simulink model "fixed_wing_sim"  (Simulink 8.7)
settings: Solver=ode4  StartTime=0.0  StopTime=T_sim  FixedStep=ts_sim  MaxStep=10e-3  RelTol=1e-3
InitFcn:
  | % Run the initialization script
  | clear all
  | aerosonde_uav_conf_model
StopFcn:
  | %show_result
  | print_results
values from neighbouring files (symbols this model uses):
  a = param(1)    [get_field.m]    (also in print_results.m = a*scale_fac/1e3; vector_field_parameters.m = 0.85)
  AilBnd = range_ail.*degrees2rad    [aerosonde_uav_conf_model.m]
  aileron_limits = [-20*pi/180;20*pi/180]    [aerosonde_uav_conf_model.m]
  AlphaBnd = range_alpha.*degrees2rad    [aerosonde_uav_conf_model.m]
  amp_theta = amp_theta*2    [vector_field_parameters.m]
  amp_theta_c = ((1/4)*[1 1 1]/6)*U_theta*tau_theta    [vector_field_parameters.m]
  amp_v_c = [1 1 1]*(tau_v*U_v)/6    [vector_field_parameters.m]
  amp_x = [5 5 5]    [vector_field_parameters.m]
  amp_y = [5 5 5]    [vector_field_parameters.m]
  amp_z = amp_z*2    [vector_field_parameters.m]
  amp_z_c = [1 1 1]*(tau_z*U_z)/6/2    [vector_field_parameters.m]
  b = param(2)    [get_field.m]    (also in print_results.m = b*scale_fac/1e3; vector_field_parameters.m = 0.08)
  BetaBnd = range_beta.*degrees2rad    [aerosonde_uav_conf_model.m]
  Bw = 2.8956    [aerosonde_uav_conf_model.m]
  c = param(3)    [get_field.m]    (also in vector_field_parameters.m = -0.13)
  CD_0 = 0.0434    [aerosonde_uav_conf_model.m]
  CD_ail = ones(length(AlphaBnd),1)*CD_aux_ail    [aerosonde_uav_conf_model.m]
  CD_alpha_beta = zeros(length(AlphaBnd),length(BetaBnd))    [aerosonde_uav_conf_model.m]
  CD_elev = ones(length(AlphaBnd),1)*CD_aux_elev    [aerosonde_uav_conf_model.m]
  CD_mind = 0.23    [aerosonde_uav_conf_model.m]
  CD_rud = ones(length(AlphaBnd),1)*CD_aux_rud    [aerosonde_uav_conf_model.m]
  CL_0 = 0.23    [aerosonde_uav_conf_model.m]
  Cl_ail = ones(length(AlphaBnd),1)*Cl_aux_ail    [aerosonde_uav_conf_model.m]
  CL_alpha_beta = CL_alpha*ones(1,length(BetaBnd))    [aerosonde_uav_conf_model.m]
  Cl_alpha_beta = ones(length(AlphaBnd),1)*Cl_beta    [aerosonde_uav_conf_model.m]
  CL_alphadot = 1.9724    [aerosonde_uav_conf_model.m]
  CL_elev = ones(length(AlphaBnd),1)*CL_aux_elev    [aerosonde_uav_conf_model.m]
  Cl_P = ones(length(AlphaBnd),1)*Cl_aux_P    [aerosonde_uav_conf_model.m]
  CL_Q = 7.9543*QBnd    [aerosonde_uav_conf_model.m]
  Cl_R = ones(length(AlphaBnd),1)*Cl_aux_R    [aerosonde_uav_conf_model.m]
  Cl_rud = ones(length(AlphaBnd),1)*Cl_aux_rud    [aerosonde_uav_conf_model.m]
  CLE_alphat = zeros(1,length(AlphaBnd))    [aerosonde_uav_conf_model.m]
  CLE_elev = 0    [aerosonde_uav_conf_model.m]
  Cm0 = 0.135    [aerosonde_uav_conf_model.m]
  Cm_alpha_beta = Cm_alpha*ones(1,length(BetaBnd))    [aerosonde_uav_conf_model.m]
  Cm_alphadot = -10.3796    [aerosonde_uav_conf_model.m]
  Cm_elev = ones(length(AlphaBnd),1)*Cm_aux_elev    [aerosonde_uav_conf_model.m]
  Cm_Q = -38.2067*QBnd    [aerosonde_uav_conf_model.m]
  Cn_ail = ones(length(AlphaBnd),1)*Cn_aux_ail    [aerosonde_uav_conf_model.m]
  Cn_alpha_beta = ones(length(AlphaBnd),1)*Cn_beta    [aerosonde_uav_conf_model.m]
  Cn_P = ones(length(AlphaBnd),1)*Cn_aux_P    [aerosonde_uav_conf_model.m]
  Cn_R = ones(length(AlphaBnd),1)*Cn_aux_R    [aerosonde_uav_conf_model.m]
  Cn_rud = ones(length(AlphaBnd),1)*Cn_aux_rud    [aerosonde_uav_conf_model.m]
  CT_save = CT_save.*10    [aerosonde_uav_conf_model.m]    (also in helice.mat = [0.115262 0.00375054783545 -0.00666475255621 -0.006665219028)
  curve = 1    [vector_field_parameters.m]
  Cw = 0.189941    [aerosonde_uav_conf_model.m]
  CY_ail = ones(length(AlphaBnd),1)*CY_aux_ail    [aerosonde_uav_conf_model.m]
  CY_alpha_beta = ones(length(AlphaBnd),1)*CY_beta    [aerosonde_uav_conf_model.m]
  CY_P = zeros(length(AlphaBnd),length(PBnd))    [aerosonde_uav_conf_model.m]
  CY_R = zeros(length(AlphaBnd),length(RBnd))    [aerosonde_uav_conf_model.m]
  CY_rud = ones(length(AlphaBnd),1)*CY_aux_rud    [aerosonde_uav_conf_model.m]
  d = param(4)    [get_field.m]    (also in vector_field_parameters.m = -0.04)
  D_hel = 0.15    [aerosonde_uav_conf_model.m]
  d_wash = 0    [aerosonde_uav_conf_model.m]
  delta_CD = 1    [aerosonde_uav_conf_model.m]
  delta_CL = 1    [aerosonde_uav_conf_model.m]
  delta_Cl = 1    [aerosonde_uav_conf_model.m]
  delta_Cm = 1    [aerosonde_uav_conf_model.m]
  delta_Cn = 1    [aerosonde_uav_conf_model.m]
  delta_CY = 1    [aerosonde_uav_conf_model.m]
  delta_FT = 1    [aerosonde_uav_conf_model.m]
  Delta_V_EH = [ 2 1.7365 1.2985 1.0890 1.0205]    [aerosonde_uav_conf_model.m]
  Delta_V_J = [ 0 0.4 0.7 1.4 2.1]    [aerosonde_uav_conf_model.m]
  elevator_limits = [-15*pi/180;15*pi/180]    [aerosonde_uav_conf_model.m]
  ElevBnd = range_elev.*degrees2rad    [aerosonde_uav_conf_model.m]
  F_T = 19    [aerosonde_uav_conf_model.m]
  f_theta = ([5 3 1]+rand(1,3))*0.05*2*pi/freq_divisor    [vector_field_parameters.m]
  f_theta_c = ([5 3 1]+rand(1,3))*0.05*2*pi/freq_divisor    [vector_field_parameters.m]
  f_v_c = ([4 2 0.5]+rand(1,3))*0.05*2*pi/freq_divisor    [vector_field_parameters.m]
  f_x = ([6 4 2]+rand(1,3))*0.05*2*pi/freq_divisor    [vector_field_parameters.m]
  f_y = ([6 4 2]+rand(1,3))*0.05*2*pi/freq_divisor    [vector_field_parameters.m]
  f_z = ([6 4 2]+rand(1,3))*0.05*2*pi/freq_divisor    [vector_field_parameters.m]
  f_z_c = ([4 2 0.5]+rand(1,3))*0.05*2*pi/freq_divisor    [vector_field_parameters.m]
  g1 = param(5)    [get_field.m]    (also in vector_field_parameters.m = 4)
  gain_G = param(6)    [get_field.m]    (also in vector_field_parameters.m = 2.5)
  gravity = 9.807    [aerosonde_uav_conf_model.m]
  H_0 = 200    [vector_field_parameters.m]
  Heq = 200    [aerosonde_uav_conf_model.m]    (also in vector_field_parameters.m)
  induced_drag = 1/(pi*AR*osw)    (= 0.0278403324809)    [aerosonde_uav_conf_model.m]
  isTrimming = 0    [aerosonde_uav_conf_model.m]
  J_save = J_save.*1.5    [aerosonde_uav_conf_model.m]    (also in helice.mat = [0 1.22229381539 1.27367709689 1.27367940534 1.27361400442 1)
  Jx = 0.7795    [aerosonde_uav_conf_model.m]
  Jxz = 0.1211    [aerosonde_uav_conf_model.m]
  Jy = 1.122    [aerosonde_uav_conf_model.m]
  Jz = 1.752    [aerosonde_uav_conf_model.m]
  KC_h = 0.28    [aerosonde_uav_conf_model.m]
  KC_phi = -1.18    [aerosonde_uav_conf_model.m]
  KC_psi = 0.03    [aerosonde_uav_conf_model.m]
  KC_r = -0.0073    [aerosonde_uav_conf_model.m]
  KC_theta = -1.1482    [aerosonde_uav_conf_model.m]
  KC_vt = 0.9948*1    (= 0.9948)    [aerosonde_uav_conf_model.m]
  KE = -0.1562    [aerosonde_uav_conf_model.m]
  Kp = 0.18    [vector_field_parameters.m]
  KR = 0.0130    (= 0.013)    [aerosonde_uav_conf_model.m]
  Ksad = param(3)    [get_field.m]    (also in print_results.m = Ksad*scale_fac/1e3; vector_field_parameters.m = 0)
  KT = 0.0792    [aerosonde_uav_conf_model.m]
  Kv = 1    [vector_field_parameters.m]
  LIM_CENTER = LIM_CENTER*scale_fac/1e3    [print_results.m]    (also in vector_field_parameters.m = 0.2)
  M = 8.5    [aerosonde_uav_conf_model.m]    (also in print_results.m = 0)
  motor_min = 0.1    [aerosonde_uav_conf_model.m]
  motor_rate = 1    [aerosonde_uav_conf_model.m]
  p_theta = rand(1,3)*2*pi    [vector_field_parameters.m]
  p_theta_c = rand(1,3)*2*pi    [vector_field_parameters.m]
  p_v_c = rand(1,3)*2*pi    [vector_field_parameters.m]
  p_x = rand(1,3)*2*pi    [vector_field_parameters.m]
  p_y = rand(1,3)*2*pi    [vector_field_parameters.m]
  p_z = rand(1,3)*2*pi    [vector_field_parameters.m]
  p_z_c = rand(1,3)*2*pi    [vector_field_parameters.m]
  PBnd = range_P.*degrees2rad    [aerosonde_uav_conf_model.m]
  perc_int_max = 0.8    [aerosonde_uav_conf_model.m]
  phi_max = 20*pi/180    (= 0.349065850399)    [aerosonde_uav_conf_model.m]
  phi_min = -20*pi/180    (= -0.349065850399)    [aerosonde_uav_conf_model.m]
  QBnd = range_Q.*degrees2rad    [aerosonde_uav_conf_model.m]
  r = sqrt(m)    [animation.m]    (also in print_results.m)
  r_aero_abc = r_aero_struct*[-1 0 0;0 1 0;0 0 -1]    [aerosonde_uav_conf_model.m]
  r_cg_abc = r_cg_struct*[-1 0 0;0 1 0;0 0 -1]    [aerosonde_uav_conf_model.m]
  r_motor_abc = r_motor_struct*[-1 0 0;0 1 0;0 0 -1]    [aerosonde_uav_conf_model.m]
  r_tail_abc = r_aero_struct*[-1 0 0;0 1 0;0 0 -1]    [aerosonde_uav_conf_model.m]
  RBnd = range_R.*degrees2rad    [aerosonde_uav_conf_model.m]
  rho = 0.1    [aerosonde_uav_conf_model.m]
  ... (+40 more)
undefined symbols (not defined in the file or in its folder): Earth, F, Light, MIL, WGS84
libraries: aerolibwind2 x2, aerolibtransform2 x2, aerolibfltsims x1, aerolibconvert2 x1, dspsigops x1
(part 2 of 3)

== system fixed_wing_sim/A/C + Low Level Control /UAV Internal Closed Loops/UAV model/Output ==
  states : Inport
  acc : Inport  Port=2
  V_WIND : Inport  Port=3
  V_NED : Inport  Port=4
  Bus Creator : BusCreator  Inputs=11
  Bus Creator4 : BusCreator  Inputs=15
  Bus Selector : BusSelector  OutputSignals=h,theta,phi,psi,R,p_N,p_E,P,Q,R
  Bus Selector1 : BusSelector  OutputSignals=x_acc,y_acc,z_acc
  Bus Selector2 : BusSelector  OutputSignals=VT
  Bus Selector3 : BusSelector  OutputSignals=vel_N,vel_E,vel_D
  Demux : Demux  Outputs=3
  Derivative : Derivative
  Gain : Gain  Gain=180/pi
  Mux : Mux  Inputs=3
  Scope : Scope  NumInputPorts=3
  Scope1 : Scope
  Scope2 : Scope
  Terminator1 : Terminator
  Trigonometric Function : Trigonometry  Operator=atan2
  rad2deg : Gain  Gain=180/pi
  rad2deg1 : Gain  Gain=180/pi
  rad2deg2 : Gain  Gain=180/pi
  Out_model : Outport
  wires:
  states/1 -> Bus Selector/1
  acc/1 -> Bus Selector1/1
  V_WIND/1 -> Bus Selector2/1
  Bus Creator/1 -> Out_model/1
  V_NED/1 -> Bus Selector3/1
  Trigonometric Function/1 -> Bus Creator4/15, Gain/1
  Bus Selector3/1 -> Bus Creator4/7, Bus Creator/8, Mux/1, Trigonometric Function/2  "<vel_N>"
  Bus Selector3/2 -> Trigonometric Function/1, Bus Creator4/8, Bus Creator/9, Mux/2  "<vel_E>"
  Bus Selector/1 -> Bus Creator/1  "<h>"
  Bus Selector/2 -> rad2deg1/1, Bus Creator4/14, Bus Creator/2  "<theta>"
  Bus Selector/3 -> rad2deg/1, Bus Creator4/13, Bus Creator/3  "<phi>"
  Bus Selector/4 -> rad2deg2/1, Bus Creator/11, Terminator1/1  "<psi>"
  Bus Selector/5 -> Bus Creator/5  "<R>"
  Bus Selector/6 -> Scope1/1, Bus Creator/6  "<p_N>"
  Bus Selector/7 -> Bus Creator/7  "<p_E>"
  Gain/1 -> Bus Creator/4  "Psi_heading"
  Bus Selector2/1 -> Bus Creator/10  "<VT>"
  rad2deg1/1 -> Scope/1
  rad2deg/1 -> Scope/2
  rad2deg2/1 -> Scope/3
  Bus Selector1/1 -> Bus Creator4/1  "<x_acc>"
  Bus Selector1/2 -> Bus Creator4/2  "<y_acc>"
  Bus Selector1/3 -> Bus Creator4/3  "<z_acc>"
  Bus Creator4/1 -> Scope2/1
  Bus Selector/8 -> Bus Creator4/4  "<P>"
  Bus Selector/9 -> Bus Creator4/5  "<Q>"
  Bus Selector/10 -> Bus Creator4/6  "<R>"
  Bus Selector3/3 -> Mux/3, Bus Creator4/9  "<vel_D>"
  Mux/1 -> Derivative/1
  Derivative/1 -> Demux/1
  Demux/1 -> Bus Creator4/10
  Demux/2 -> Bus Creator4/11
  Demux/3 -> Bus Creator4/12

== system fixed_wing_sim/A/C + Low Level Control /UAV Internal Closed Loops/UAV model/Servos ==
  control : Inport
  Bus Creator : BusCreator  Inputs=3
  Bus Selector : BusSelector  OutputSignals=elevator,aileron,rudder,throttle
  Gain{,1..3} (4 alike) : Gain  Gain=180/pi
  Saturation : Saturate  UpperLimit=1  LowerLimit=motor_min
  Saturation1 : Saturate  UpperLimit=elevator_limits(2)  LowerLimit=elevator_limits(1)
  Saturation2 : Saturate  UpperLimit=rudder_limits(2)  LowerLimit=rudder_limits(1)
  Saturation3 : Saturate  UpperLimit=aileron_limits(2)  LowerLimit=aileron_limits(1)
  Scope : Scope  NumInputPorts=4
  angle_servos : Outport
  th_servo : Outport  Port=2
  wires:
  Saturation3/1 -> Bus Creator/2, Gain1/1  "aileron"
  Bus Creator/1 -> angle_servos/1
  Saturation1/1 -> Gain/1, Bus Creator/1  "elevator"
  Saturation2/1 -> Gain2/1, Bus Creator/3  "rudder"
  Saturation/1 -> Gain3/1, th_servo/1  "throttle"
  control/1 -> Bus Selector/1
  Bus Selector/4 -> Saturation/1  "<throttle>"
  Bus Selector/1 -> Saturation1/1  "<elevator>"
  Bus Selector/2 -> Saturation3/1  "<aileron>"
  Bus Selector/3 -> Saturation2/1  "<rudder>"
  Gain/1 -> Scope/1
  Gain3/1 -> Scope/4
  Gain2/1 -> Scope/3
  Gain1/1 -> Scope/2

== system fixed_wing_sim/A/C + Low Level Control /UAV Internal Closed Loops/UAV model/Aerodynamics Equations/F_Aero_WIND ==
  v_WIND : Inport
  servos : Inport  Port=2
  density : Inport  Port=3
  w_ABC : Inport  Port=4
  Bus Creator : BusCreator  Inputs=3
  Bus Selector : BusSelector  OutputSignals=VT,alpha,beta
  Bus Selector2 : BusSelector  OutputSignals=P,Q,R
  Drag Force : Subsystem
  Gain : Gain  Gain=-1
  Gain1 : Gain  Gain=-1
  Gain2 : Gain
  Lift Force : Subsystem
  Side Force : Subsystem
  F_WIND : Outport
  wires:
  Drag Force/1(D) -> Gain/1
  Bus Creator/1 -> F_WIND/1
  v_WIND/1 -> Bus Selector/1
  Gain/1 -> Bus Creator/1
  Bus Selector/1 -> Side Force/3(VT), Lift Force/3(VT), Drag Force/4(VT)  "<VT>"
  Bus Selector/2 -> Drag Force/1(alpha), Lift Force/1(alpha), Side Force/2(alpha)  "<alpha>"
  Side Force/1(Y) -> Gain2/1
  Gain1/1 -> Bus Creator/3
  density/1 -> Side Force/4(density), Drag Force/5(density), Lift Force/4(density)
  Bus Selector/3 -> Drag Force/2(beta), Side Force/1(beta), Lift Force/2(beta)  "<beta>"
  w_ABC/1 -> Bus Selector2/1
  Lift Force/1(L) -> Gain1/1
  Bus Selector2/1 -> Side Force/6(P)  "<P>"
  Bus Selector2/2 -> Lift Force/6(Q)  "<Q>"
  Bus Selector2/3 -> Side Force/7(R)  "<R>"
  Gain2/1 -> Bus Creator/2
  servos/1 -> Side Force/5(servos), Lift Force/5(servos), Drag Force/6(servos)
  Lift Force/2(CL) -> Drag Force/3(CL)

== system fixed_wing_sim/A/C + Low Level Control /UAV Internal Closed Loops/UAV model/Aerodynamics Equations/F_TAIL_WIND --> F_ABC ==
  note: ABC = ( R_(alpha) )^T * WIND
  v_WIND : Inport
  WIND : Inport  Port=2
  Bus Selector : BusSelector  OutputSignals=alpha_t
  Math Function : Math  Operator=transpose  SaturateOnIntegerOverflow=on
  Product1 : Product  Multiplication=Matrix(*)  RndMeth=Zero
  R_(alpha) : Subsystem
  ABC : Outport
  wires:
  v_WIND/1 -> Bus Selector/1
  WIND/1 -> Product1/2
  Product1/1 -> ABC/1
  Math Function/1 -> Product1/1
  Bus Selector/1 -> R_(alpha)/1(In1)  "<alpha_t>"
  R_(alpha)/1(Out1) -> Math Function/1

== system fixed_wing_sim/A/C + Low Level Control /UAV Internal Closed Loops/UAV model/Aerodynamics Equations/F_Tail_WIND ==
  note: Dynamic Pressure
  v_WIND : Inport
  servos : Inport  Port=2
  density : Inport  Port=3
  Delta_V_EH : Inport  Port=4
  teste_V : Inport  Port=5
  Add : Sum
  Area Empenagem : Gain  Gain=Sh
  Bus Selector : BusSelector  OutputSignals=alpha_t,VT_tail
  Bus Selector1 : BusSelector  OutputSignals=elevator
  Bus Selector2 : BusSelector  OutputSignals=VT
  CLE_alphat : Lookup  InputValues=AlphaBnd  Table=CLE_alphat
  Constant4 : Constant  Value=0
  Gain : Gain  Gain=0.5
  Gain3 : Gain  Gain=CLE_elev  SaturateOnIntegerOverflow=on  OutDataTypeStr=Inherit: Same as input  ParamDataTypeStr=Inherit: Same as input
  Math Function : Math  Operator=square  SaturateOnIntegerOverflow=on
  Mux : Mux  Inputs=3
  Product : Product  RndMeth=Zero
  Product1 : Product  RndMeth=Zero
  Product2 : Product  RndMeth=Zero
  Terminator : Terminator
  Z + down : Gain  Gain=-1
  F_Tail_WIND : Outport
  wires:
  v_WIND/1 -> Bus Selector/1
  servos/1 -> Bus Selector1/1
  Bus Selector1/1 -> Gain3/1  "<elevator>"
  Bus Selector/1 -> CLE_alphat/1  "<alpha_t>"
  Product/1 -> Gain/1
  density/1 -> Product/1
  Math Function/1 -> Product/2
  Product1/1 -> Math Function/1
  Delta_V_EH/1 -> Product1/2
  CLE_alphat/1 -> Add/1
  Gain3/1 -> Add/2
  Add/1 -> Product2/1
  Gain/1 -> Product2/2
  Product2/1 -> Area Empenagem/1
  Mux/1 -> F_Tail_WIND/1
  Area Empenagem/1 -> Z + down/1
  Z + down/1 -> Mux/3
  Constant4/1 -> Mux/1, Mux/2
  teste_V/1 -> Bus Selector2/1
  Bus Selector/2 -> Product1/1  "<VT_tail>"
  Bus Selector2/1 -> Terminator/1  "<VT>"

== system fixed_wing_sim/A/C + Low Level Control /UAV Internal Closed Loops/UAV model/Aerodynamics Equations/F_WIND --> F_ABC ==
  note: ABC = ( R_beta * R_(alpha) )^T * WIND
  v_WIND : Inport
  WIND : Inport  Port=2
  Bus Selector : BusSelector  OutputSignals=alpha,beta
  Math Function : Math  Operator=transpose  SaturateOnIntegerOverflow=on
  Product : Product  Multiplication=Matrix(*)  RndMeth=Zero
  Product1 : Product  Multiplication=Matrix(*)  RndMeth=Zero
  R_(alpha) : Subsystem
  R_beta : Subsystem
  ABC : Outport
  wires:
  R_beta/1(Out1) -> Product/1
  R_(alpha)/1(Out1) -> Product/2
  v_WIND/1 -> Bus Selector/1
  WIND/1 -> Product1/2
  Product1/1 -> ABC/1
  Product/1 -> Math Function/1
  Math Function/1 -> Product1/1
  Bus Selector/1 -> R_(alpha)/1(In1)  "<alpha>"
  Bus Selector/2 -> R_beta/1(In1)  "<beta>"

== system fixed_wing_sim/A/C + Low Level Control /UAV Internal Closed Loops/UAV model/Aerodynamics Equations/M_Aero_WIND ==
  v_WIND : Inport
  servos : Inport  Port=2
  density : Inport  Port=3
  w_ABC : Inport  Port=4
  Bus Creator : BusCreator  Inputs=3
  Bus Selector : BusSelector  OutputSignals=VT,alpha,beta
  Bus Selector2 : BusSelector  OutputSignals=P,Q,R
  Pitching Moment : Subsystem
  Rolling Moment : Subsystem
  Yawing Moment : Subsystem
  M_ABC : Outport
  wires:
  Bus Creator/1 -> M_ABC/1
  v_WIND/1 -> Bus Selector/1
  servos/1 -> Rolling Moment/7(servos), Pitching Moment/5(servo), Yawing Moment/5(servos)
  w_ABC/1 -> Bus Selector2/1
  density/1 -> Yawing Moment/4(density), Rolling Moment/4(density), Pitching Moment/4(density)
  Rolling Moment/1(Cl) -> Bus Creator/1
  Pitching Moment/1(Cm) -> Bus Creator/2
  Yawing Moment/1(Cn) -> Bus Creator/3
  Bus Selector2/1 -> Rolling Moment/5(P), Yawing Moment/6(P)  "<P>"
  Bus Selector2/2 -> Pitching Moment/6(Q)  "<Q>"
  Bus Selector2/3 -> Yawing Moment/7(R), Rolling Moment/6(R)  "<R>"
  Bus Selector/1 -> Rolling Moment/3(VT), Yawing Moment/3(VT), Pitching Moment/3(VT)  "<VT>"
  Bus Selector/3 -> Rolling Moment/1(beta), Yawing Moment/1(beta), Pitching Moment/2(beta)  "<beta>"
  Bus Selector/2 -> Rolling Moment/2(alpha), Pitching Moment/1(alpha), Yawing Moment/2(alpha)  "<alpha>"

== system fixed_wing_sim/A/C + Low Level Control /UAV Internal Closed Loops/UAV model/Aerodynamics Equations/U' V' W' --> VT,alpha,beta ==
  v_ABC : Inport
  Bus Creator : BusCreator  Inputs=3
  alpha : Fcn  Expr=atan2(u(3),u(1))
  beta : Fcn  Expr=asin(u(2)/sqrt(u(1)^2 + u(2)^2 + u(3)^2))
  vector_norm : Fcn  Expr=sqrt(u(1)^2 + u(2)^2 + u(3)^2)
  v_WIND : Outport
  wires:
  Bus Creator/1 -> v_WIND/1
  v_ABC/1 -> vector_norm/1, alpha/1, beta/1
  vector_norm/1 -> Bus Creator/1  "VT"
  alpha/1 -> Bus Creator/2  "alpha"
  beta/1 -> Bus Creator/3  "beta"

== system fixed_wing_sim/A/C + Low Level Control /UAV Internal Closed Loops/UAV model/Aerodynamics Equations/U' V' W' --> Vtail, alpha_t ==
  v_ABC : Inport
  w_ABC : Inport  Port=2
  wind : Inport  Port=3
  Add : Sum  Inputs=++-
  Bus Creator : BusCreator  Inputs=2
  Bus Selector : BusSelector  OutputSignals=U,W
  Bus Selector1 : BusSelector  OutputSignals=Q
  Bus Selector2 : BusSelector  OutputSignals=alpha,VT
  Constant1 : Constant  Value=xt
  Gain : Gain  Gain=d_wash
  Mux : Mux  Inputs=2
  Product : Product  RndMeth=Zero
  Product1 : Product  RndMeth=Zero
  VT_tail : Fcn  Expr=sqrt(u(1)^2 + u(2)^2 )
  alpha_t : Fcn  Expr=atan2(u(2),u(1))
  v_TAIL : Outport
  wires:
  Bus Creator/1 -> v_TAIL/1
  VT_tail/1 -> Bus Creator/1  "VT_tail"
  alpha_t/1 -> Bus Creator/2  "alpha_t"
  v_ABC/1 -> Bus Selector/1
  w_ABC/1 -> Bus Selector1/1
  Bus Selector1/1 -> Product/1  "<Q>"
  Constant1/1 -> Product/2
  Bus Selector/2 -> Add/1  "<W>"
  Product/1 -> Add/2
  Bus Selector/1 -> Mux/1  "<U>"
  Add/1 -> Mux/2
  Mux/1 -> VT_tail/1, alpha_t/1
  Gain/1 -> Product1/1
  wind/1 -> Bus Selector2/1
  Bus Selector2/1 -> Gain/1  "<alpha>"
  Bus Selector2/2 -> Product1/2  "<VT>"
  Product1/1 -> Add/3

== system fixed_wing_sim/A/C + Low Level Control /UAV Internal Closed Loops/UAV model/Atmosphere Model/Standard Atmosphere ==
  var_states : Inport
  g : Inport  Port=2
  Altitude Equilibrio : Constant  Value=Heq
  Bus Selector : BusSelector  OutputSignals=h
  Calc. Density : Fcn  Expr=1.225*(u(1)/288.15)^(-u(2)/(-0.0065*287.04)-1)
  Calc. Pressure : Fcn  Expr=101325*(u(1)/288.15)^(-u(2)/(-0.0065*287.04))
  Calc. Temperatura : Fcn  Expr=288.15 -0.0065*u(1)
  Function for Sound Speed : Fcn  Expr=sqrt(u*1.4*287.04)
  Mux : Mux  Inputs=2
  Mux1 : Mux  Inputs=2
  Terminator : Terminator
  rho (kg/m3) : Outport
  a (m/s) : Outport  Port=2
  T (K) : Outport  Port=3
  P (N/m2) : Outport  Port=4
  wires:
  g/1 -> Mux1/2, Mux/2
  Mux/1 -> Calc. Temperatura/1
  Mux1/1 -> Calc. Pressure/1, Calc. Density/1
  Calc. Temperatura/1 -> Mux1/1, Function for Sound Speed/1, T (K)/1  "temperature (K)"
  Calc. Pressure/1 -> P (N/m2)/1  "pressure (Pa)"
  Calc. Density/1 -> rho (kg/m3)/1  "density (Kg/m3)"
  Function for Sound Speed/1 -> a (m/s)/1  "sound speed (m/s)"
  var_states/1 -> Bus Selector/1
  Altitude Equilibrio/1 -> Terminator/1
  Bus Selector/1 -> Mux/1  "<h>"

== system fixed_wing_sim/A/C + Low Level Control /UAV Internal Closed Loops/UAV model/Body-Axes 6DOF Equations/Force Equations ==
  note: Gravity Vector in ABC
  note: Forces in ABC
  note: Term due derivative had token in NED but
      | velocity in ABC
  note: Equation: v_ABC_dot = (1/m) * F_A,T + R_ned_abc * gravity - w_ABC x v_ABC
  F_Aero_ABC : Inport
  attitude : Inport  Port=2
  F_Thrust_ABC : Inport  Port=3
  w_ABC : Inport  Port=4
  v_ABC : Inport  Port=5
  F_tail_ABC : Inport  Port=6
  Add : Sum  Inputs=+++
  Add1 : Sum  Inputs=++-
  Bus Creator : BusCreator  Inputs=3
  Demux : Demux  Outputs=3
  Mux : Mux  Inputs=3
  NED --> ABC : Subsystem
  Product : Product  RndMeth=Zero
  Vector Product : Subsystem  Description=Vector Product
  axis_X : Constant  Value=0
  axis_Y : Constant  Value=0
  axis_Z : Constant  Value=gravity
  inv_M : Constant  Value=1/M
  v_ABC_dot : Outport
  acc_x_y_z : Outport  Port=2
  wires:
  axis_X/1 -> Mux/1
  axis_Y/1 -> Mux/2
  axis_Z/1 -> Mux/3
  Mux/1 -> NED --> ABC/2(NED)
  F_Aero_ABC/1 -> Add/1
  F_Thrust_ABC/1 -> Add/2
  Add/1 -> Product/1
  inv_M/1 -> Product/2
  attitude/1 -> NED --> ABC/1(attitude)
  w_ABC/1 -> Vector Product/1(V1)
  v_ABC/1 -> Vector Product/2(V2)
  Product/1 -> Add1/1, Demux/1
  Vector Product/1(V1 x V2) -> Add1/3
  Add1/1 -> v_ABC_dot/1
  NED --> ABC/1(ABC) -> Add1/2
  Bus Creator/1 -> acc_x_y_z/1
  Demux/1 -> Bus Creator/1  "x_acc"
  Demux/2 -> Bus Creator/2  "y_acc"
  Demux/3 -> Bus Creator/3  "z_acc"
  F_tail_ABC/1 -> Add/3

== system fixed_wing_sim/A/C + Low Level Control /UAV Internal Closed Loops/UAV model/Body-Axes 6DOF Equations/Kinematic Equations ==
  note: phi_dot     = P + Q*tan(theta)*sin(phi) + R*tan(theta)*cos(phi)
      |          theta_dot =  Q*cos(phi) - R*sin(phi)
      |                           psi_dot     = (Q*sin(phi) + R*cos(phi)) / cos (theta)
  note: Relationship between angular velocity of Euler angles (phi_dot, theta_dot, psi_dot) and angular velocity of axis ABC (P,Q,R)
  attitude : Inport
  w_ABC : Inport  Port=2
  Bus Selector : BusSelector  OutputSignals=phi,theta,psi
  Bus Selector1 : BusSelector  OutputSignals=P,Q,R
  Mux : Mux  Inputs=3
  Product{,1..4,6..7} (7 alike) : Product  SaturateOnIntegerOverflow=on  OutDataTypeStr=Inherit: Same as first input
  Product5 : Product  Inputs=/*  SaturateOnIntegerOverflow=on  OutDataTypeStr=Inherit: Same as first input
  Sum1 : Sum  SaturateOnIntegerOverflow=on
  Sum2 : Sum  SaturateOnIntegerOverflow=on
  Sum3 : Sum  Inputs=+-  SaturateOnIntegerOverflow=on
  Sum4 : Sum  SaturateOnIntegerOverflow=on
  Terminator : Terminator
  cos (phi) : Trigonometry  Operator=cos
  cos (theta) : Trigonometry  Operator=cos
  sin (phi) : Trigonometry
  tan (theta) : Trigonometry  Operator=tan
  attitude_dot : Outport
  wires:
  Bus Selector/2 -> cos (theta)/1, tan (theta)/1  "<theta>"
  Bus Selector/1 -> cos (phi)/1, sin (phi)/1  "<phi>"
  sin (phi)/1 -> Product/1, Product4/1, Product6/1
  cos (phi)/1 -> Product1/1, Product3/1, Product7/1
  Product1/1 -> Sum1/1
  Product/1 -> Sum1/2
  Sum1/1 -> Product2/1
  Product2/1 -> Sum2/1
  Sum2/1 -> Mux/1
  Bus Selector/3 -> Terminator/1  "<psi>"
  Product3/1 -> Sum3/1
  w_ABC/1 -> Bus Selector1/1
  Product4/1 -> Sum3/2
  cos (theta)/1 -> Product5/1
  Product6/1 -> Sum4/1
  Product7/1 -> Sum4/2
  Sum4/1 -> Product5/2
  Sum3/1 -> Mux/2
  Product5/1 -> Mux/3
  Bus Selector1/1 -> Sum2/2  "<P>"
  Mux/1 -> attitude_dot/1
  Bus Selector1/2 -> Product/2, Product3/2, Product6/2  "<Q>"
  Bus Selector1/3 -> Product1/2, Product4/2, Product7/2  "<R>"
  tan (theta)/1 -> Product2/2
  attitude/1 -> Bus Selector/1

== system fixed_wing_sim/A/C + Low Level Control /UAV Internal Closed Loops/UAV model/Body-Axes 6DOF Equations/Moment Equations ==
  note: Term due derivative had token in NED but
      | angular velocity in ABC
  note: Equation: w_ABC_dot = J^(-1)*[ M_A,T - w_ABC x J * w_ABC ]
  note: Moments in ABC due position of motor and aerodynamics
      | forces em relação gravity center and aerodynamics moments
  M_Aero_ABC : Inport
  F_Thrust_ABC : Inport  Port=2
  w_ABC : Inport  Port=3
  F_Aero_ABC : Inport  Port=4
  F_tail_ABC : Inport  Port=5
  Add : Sum  Inputs=+-
  Add1 : Sum  Inputs=-+
  Add2 : Sum  Inputs=-+
  C.G. position : Constant  Value=r_cg_abc
  Engine position1 : Constant  Value=r_aero_abc
  Engine position2 : Constant  Value=r_tail_abc
  Inertia : Subsystem
  Inverse Inertia Matrix : Subsystem
  Motor position : Constant  Value=r_motor_abc
  Product : Product  Multiplication=Matrix(*)  SaturateOnIntegerOverflow=on  OutDataTypeStr=Inherit: Same as first input
  Product1 : Product  Multiplication=Matrix(*)  SaturateOnIntegerOverflow=on  OutDataTypeStr=Inherit: Same as first input
  Product2 : Product  Multiplication=Matrix(*)  SaturateOnIntegerOverflow=on  OutDataTypeStr=Inherit: Same as first input
  Produto Vetorial1 : Subsystem
  Produto Vetorial2 : Subsystem
  Produto Vetorial3 : Subsystem
  Produto Vetorial4 : Subsystem
  Sum2 : Sum  Inputs=++++  SaturateOnIntegerOverflow=on
  Sum3 : Sum  Inputs=|+-  SaturateOnIntegerOverflow=on
  w_ABC_dot : Outport
  wires:
  Inverse Inertia Matrix/1(inv J_b) -> Product/1, Product2/1
  Sum2/1 -> Product/2
  Product/1 -> Sum3/1
  Inertia/1(J_b) -> Product1/1
  w_ABC/1 -> Product1/2, Produto Vetorial1/1(V1)
  Product1/1 -> Produto Vetorial1/2(V2)
  Produto Vetorial1/1(V1 x V2) -> Product2/2
  Product2/1 -> Sum3/2
  Motor position/1 -> Add/1
  F_Thrust_ABC/1 -> Produto Vetorial2/2(V2)
  Sum3/1 -> w_ABC_dot/1
  F_Aero_ABC/1 -> Produto Vetorial3/2(V2)
  Produto Vetorial2/1(V1 x V2) -> Sum2/1
  M_Aero_ABC/1 -> Sum2/2
  Produto Vetorial3/1(V1 x V2) -> Sum2/3
  C.G. position/1 -> Add/2, Add1/1, Add2/1
  Add/1 -> Produto Vetorial2/1(V1)
  Engine position1/1 -> Add1/2
  Add1/1 -> Produto Vetorial3/1(V1)
  Engine position2/1 -> Add2/2
  Add2/1 -> Produto Vetorial4/1(V1)
  F_tail_ABC/1 -> Produto Vetorial4/2(V2)
  Produto Vetorial4/1(V1 x V2) -> Sum2/4

== system fixed_wing_sim/A/C + Low Level Control /UAV Internal Closed Loops/UAV model/Body-Axes 6DOF Equations/NED --> ABC ==
  note: ABC = (R_phi * R_theta * R_psi)* NED
  attitude : Inport
  v_NED : Inport  Port=2
  Bus Selector : BusSelector  OutputSignals=phi,theta,psi
  Product : Product  Multiplication=Matrix(*)  RndMeth=Zero
  Product1 : Product  Multiplication=Matrix(*)  RndMeth=Zero
  Product2 : Product  Multiplication=Matrix(*)  RndMeth=Zero
  "R_phi " : Subsystem
  R_psi : Subsystem
  R_theta : Subsystem
  v_ABC_tub : Outport
  wires:
  attitude/1 -> Bus Selector/1
  R_theta/1(Out1) -> Product/2
  Product/1 -> Product1/1
  "R_phi "/1(Out1) -> Product/1
  R_psi/1(Out1) -> Product1/2
  v_NED/1 -> Product2/2
  Product2/1 -> v_ABC_tub/1
  Product1/1 -> Product2/1
  Bus Selector/2 -> R_theta/1(In1)  "<theta>"
  Bus Selector/3 -> R_psi/1(In1)  "<psi>"
  Bus Selector/1 -> "R_phi "/1(In1)  "<phi>"

== system fixed_wing_sim/A/C + Low Level Control /UAV Internal Closed Loops/UAV model/Body-Axes 6DOF Equations/Navigation Equations ==
  note: Z + downward
  v_ABC : Inport
  attitude : Inport  Port=2
  ABC --> NED : Subsystem
  Bus Creator4 : BusCreator  Inputs=3
  Constant : Constant  Value=0  VectorParams1D=off
  Constant1 : Constant  Value=isTrimming  VectorParams1D=off
  Demux : Demux  Outputs=3
  Gain : Gain  Gain=-1
  Mux : Mux  Inputs=3
  Scope : Scope
  Scope1 : Scope
  Switch : Switch  Threshold=0.5  SaturateOnIntegerOverflow=on
  Switch1 : Switch  Threshold=0.5  SaturateOnIntegerOverflow=on
  v_NED : Outport
  v_NED_x_y : Outport  Port=2
  wires:
  attitude/1 -> ABC --> NED/1(attitude)
  v_ABC/1 -> ABC --> NED/2(v_ABC)
  Demux/3 -> Bus Creator4/3, Gain/1  "vel_D"
  ABC --> NED/1(NED) -> Demux/1
  Mux/1 -> Scope1/1, v_NED/1
  Gain/1 -> Mux/3
  Switch/1 -> Mux/1
  Switch1/1 -> Mux/2
  Constant/1 -> Switch/1, Switch1/1
  Constant1/1 -> Switch/2, Switch1/2
  Demux/1 -> Switch/3, Bus Creator4/1  "vel_N"
  Demux/2 -> Switch1/3, Bus Creator4/2  "vel_E"
  Bus Creator4/1 -> Scope/1, v_NED_x_y/1

== system fixed_wing_sim/A/C + Low Level Control /UAV Internal Closed Loops/UAV model/Aerodynamics Equations/F_Aero_WIND/Drag Force ==
  note: Dynamic Pressure
  alpha : Inport
  beta : Inport  Port=2
  CL : Inport  Port=3
  VT : Inport  Port=4
  density : Inport  Port=5
  servos : Inport  Port=6
  Add : Sum  Inputs=++++++
  Add1 : Sum  Inputs=+-
  Bus Selector1 : BusSelector  OutputSignals=elevator,aileron,rudder
  CD alpha ail : Lookup_n-D  BreakpointsForDimension1=AlphaBnd  BreakpointsForDimension2=AilBnd  Table=CD_ail  RndMeth=Simplest  InputSameDT=on
  CD alpha beta : Lookup_n-D  BreakpointsForDimension1=AlphaBnd  BreakpointsForDimension2=BetaBnd  Table=CD_alpha_beta  RndMeth=Simplest  InputSameDT=on
  CD alpha elev : Lookup_n-D  BreakpointsForDimension1=AlphaBnd  BreakpointsForDimension2=ElevBnd  Table=CD_elev  RndMeth=Simplest  InputSameDT=on
  CD alpha rud : Lookup_n-D  BreakpointsForDimension1=AlphaBnd  BreakpointsForDimension2=RudBnd  Table=CD_rud  RndMeth=Simplest  InputSameDT=on
  CD_0 : Constant  Value=CD_0
  Constant1 : Constant  Value=induced_drag
  Constant4 : Constant  Value=CD_mind
  Gain : Gain  Gain=0.5
  Math : Math  Operator=square  SaturateOnIntegerOverflow=on
  Math Function : Math  Operator=square  SaturateOnIntegerOverflow=on
  Product : Product  RndMeth=Zero
  Product1 : Product  RndMeth=Zero
  Product2 : Product  RndMeth=Zero
  Wing Area : Gain  Gain=Sw
  uncertain CD : Gain  Gain=delta_CD
  D : Outport
  wires:
  VT/1 -> Math Function/1
  Math Function/1 -> Product/1
  density/1 -> Product/2
  Wing Area/1 -> D/1
  Product/1 -> Gain/1
  Add/1 -> uncertain CD/1
  Product2/1 -> Wing Area/1
  Gain/1 -> Product2/2
  CD_0/1 -> Add/1
  servos/1 -> Bus Selector1/1
  uncertain CD/1 -> Product2/1
  CL/1 -> Add1/1
  alpha/1 -> CD alpha beta/1, CD alpha elev/1, CD alpha ail/1, CD alpha rud/1
  beta/1 -> CD alpha beta/2
  CD alpha beta/1 -> Add/2
  Bus Selector1/3 -> CD alpha rud/2  "<rudder>"
  CD alpha rud/1 -> Add/5
  CD alpha elev/1 -> Add/3
  Bus Selector1/1 -> CD alpha elev/2  "<elevator>"
  Bus Selector1/2 -> CD alpha ail/2  "<aileron>"
  CD alpha ail/1 -> Add/4
  Constant4/1 -> Add1/2
  Add1/1 -> Math/1
  Constant1/1 -> Product1/2
  Math/1 -> Product1/1
  Product1/1 -> Add/6

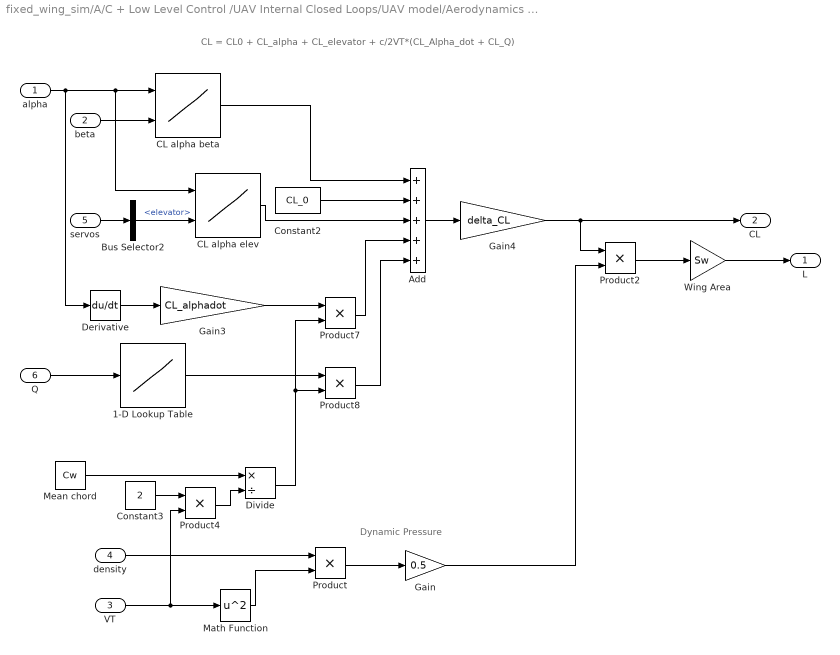
== system fixed_wing_sim/A/C + Low Level Control /UAV Internal Closed Loops/UAV model/Aerodynamics Equations/F_Aero_WIND/Lift Force ==
  note: CL = CL0 + CL_alpha + CL_elevator + c/2VT*(CL_Alpha_dot + CL_Q)
  note: Dynamic Pressure
  alpha : Inport
  beta : Inport  Port=2
  VT : Inport  Port=3
  density : Inport  Port=4
  servos : Inport  Port=5
  Q : Inport  Port=6
  1-D Lookup Table : Lookup_n-D  NumberOfTableDimensions=1  BreakpointsForDimension1=QBnd  Table=CL_Q  RndMeth=Simplest  InputSameDT=on
  Add : Sum  Inputs=+++++
  Bus Selector2 : BusSelector  OutputSignals=elevator
  CL alpha beta : Lookup_n-D  BreakpointsForDimension1=AlphaBnd  BreakpointsForDimension2=BetaBnd  Table=CL_alpha_beta  RndMeth=Simplest  InputSameDT=on
  CL alpha elev : Lookup_n-D  BreakpointsForDimension1=AlphaBnd  BreakpointsForDimension2=ElevBnd  Table=CL_elev  RndMeth=Simplest  InputSameDT=on
  Constant2 : Constant  Value=CL_0
  Constant3 : Constant  Value=2
  Derivative : Derivative
  Divide : Product  Inputs=*/
  Gain : Gain  Gain=0.5
  Gain3 : Gain  Gain=CL_alphadot
  Gain4 : Gain  Gain=delta_CL
  Math Function : Math  Operator=square  SaturateOnIntegerOverflow=on
  Mean chord : Constant  Value=Cw
  Product{,2,4,7..8} (5 alike) : Product  RndMeth=Zero
  Wing Area : Gain  Gain=Sw
  L : Outport
  CL : Outport  Port=2
  wires:
  VT/1 -> Math Function/1, Product4/2
  Wing Area/1 -> L/1
  Product/1 -> Gain/1
  alpha/1 -> Derivative/1, CL alpha beta/1, CL alpha elev/1
  Product2/1 -> Wing Area/1
  density/1 -> Product/1
  Math Function/1 -> Product/2
  Product4/1 -> Divide/2
  Mean chord/1 -> Divide/1
  Constant3/1 -> Product4/1
  Divide/1 -> Product8/2, Product7/2
  Gain/1 -> Product2/2
  Add/1 -> Gain4/1
  Constant2/1 -> Add/2
  servos/1 -> Bus Selector2/1
  Bus Selector2/1 -> CL alpha elev/2  "<elevator>"
  CL alpha elev/1 -> Add/3
  Derivative/1 -> Gain3/1
  Gain3/1 -> Product7/1
  1-D Lookup Table/1 -> Product8/1
  Q/1 -> 1-D Lookup Table/1
  Product7/1 -> Add/4
  Product8/1 -> Add/5
  Gain4/1 -> Product2/1, CL/1
  beta/1 -> CL alpha beta/2
  CL alpha beta/1 -> Add/1

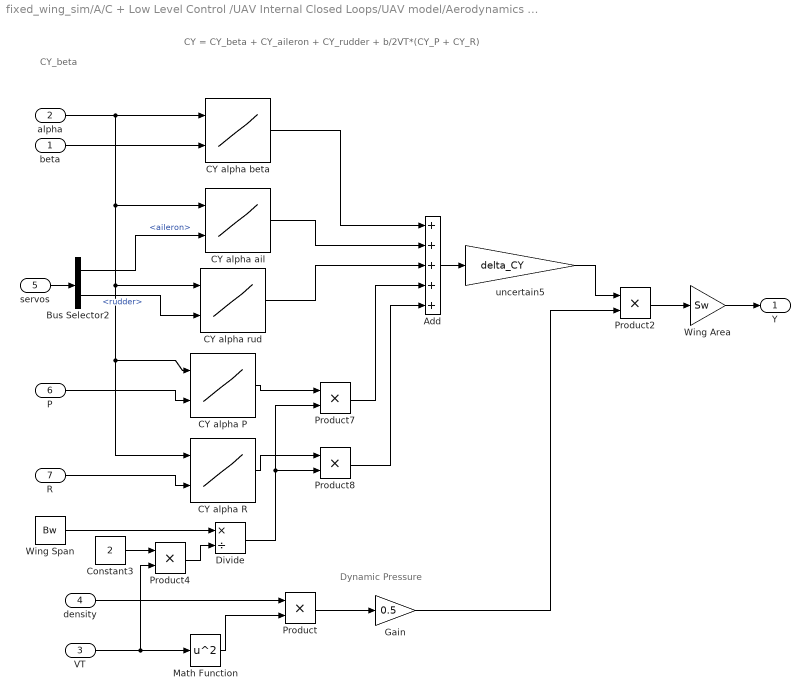
== system fixed_wing_sim/A/C + Low Level Control /UAV Internal Closed Loops/UAV model/Aerodynamics Equations/F_Aero_WIND/Side Force ==
  note: CY = CY_beta + CY_aileron + CY_rudder + b/2VT*(CY_P + CY_R)
  note: CY_beta
  note: Dynamic Pressure
  beta : Inport
  alpha : Inport  Port=2
  VT : Inport  Port=3
  density : Inport  Port=4
  servos : Inport  Port=5
  P : Inport  Port=6
  R : Inport  Port=7
  Add : Sum  Inputs=+++++
  Bus Selector2 : BusSelector  OutputSignals=aileron,rudder
  CY alpha P : Lookup_n-D  BreakpointsForDimension1=AlphaBnd  BreakpointsForDimension2=PBnd  Table=CY_P  RndMeth=Simplest  InputSameDT=on
  CY alpha R : Lookup_n-D  BreakpointsForDimension1=AlphaBnd  BreakpointsForDimension2=RBnd  Table=CY_R  RndMeth=Simplest  InputSameDT=on
  CY alpha ail : Lookup_n-D  BreakpointsForDimension1=AlphaBnd  BreakpointsForDimension2=AilBnd  Table=CY_ail  RndMeth=Simplest  InputSameDT=on
  CY alpha beta : Lookup_n-D  BreakpointsForDimension1=AlphaBnd  BreakpointsForDimension2=BetaBnd  Table=CY_alpha_beta  RndMeth=Simplest  InputSameDT=on
  CY alpha rud : Lookup_n-D  BreakpointsForDimension1=AlphaBnd  BreakpointsForDimension2=RudBnd  Table=CY_rud  RndMeth=Simplest  InputSameDT=on
  Constant3 : Constant  Value=2
  Divide : Product  Inputs=*/
  Gain : Gain  Gain=0.5
  Math Function : Math  Operator=square  SaturateOnIntegerOverflow=on
  Product{,2,4,7..8} (5 alike) : Product  RndMeth=Zero
  Wing Area : Gain  Gain=Sw
  Wing Span : Constant  Value=Bw
  uncertain5 : Gain  Gain=delta_CY
  Y : Outport
  wires:
  VT/1 -> Math Function/1, Product4/2
  Wing Area/1 -> Y/1
  Product/1 -> Gain/1
  Add/1 -> uncertain5/1
  Product2/1 -> Wing Area/1
  density/1 -> Product/1
  Math Function/1 -> Product/2
  Product4/1 -> Divide/2
  Wing Span/1 -> Divide/1
  Constant3/1 -> Product4/1
  Divide/1 -> Product8/2, Product7/2
  Product8/1 -> Add/5
  Gain/1 -> Product2/2
  Bus Selector2/2 -> CY alpha rud/2  "<rudder>"
  servos/1 -> Bus Selector2/1
  Product7/1 -> Add/4
  P/1 -> CY alpha P/2
  CY alpha P/1 -> Product7/1
  R/1 -> CY alpha R/2
  CY alpha R/1 -> Product8/1
  CY alpha ail/1 -> Add/2
  uncertain5/1 -> Product2/1
  alpha/1 -> CY alpha beta/1, CY alpha ail/1, CY alpha P/1, CY alpha R/1, CY alpha rud/1
  beta/1 -> CY alpha beta/2
  Bus Selector2/1 -> CY alpha ail/2  "<aileron>"
  CY alpha beta/1 -> Add/1
  CY alpha rud/1 -> Add/3

== system fixed_wing_sim/A/C + Low Level Control /UAV Internal Closed Loops/UAV model/Aerodynamics Equations/F_TAIL_WIND --> F_ABC/R_(alpha) ==
  note: cos  0  sin
      | 0    1    0
      | -sin   0  cos
  note: R_(alpha) -->
  In1 : Inport
  Constant : Constant
  Constant1 : Constant  Value=0
  Gain : Gain  Gain=-1
  Gain1 : Gain
  Matrix Concatenate : Concatenate  NumInputs=3  Mode=Multidimensional array
  Matrix Concatenate1 : Concatenate  NumInputs=3  Mode=Multidimensional array
  Matrix Concatenate2 : Concatenate  NumInputs=3  Mode=Multidimensional array
  Matrix Concatenate3 : Concatenate  NumInputs=3  Mode=Multidimensional array  ConcatenateDimension=2
  cos(alpha) : Trigonometry  Operator=cos
  sin(alpha) : Trigonometry
  Out1 : Outport
  wires:
  Matrix Concatenate/1 -> Matrix Concatenate3/1
  Matrix Concatenate1/1 -> Matrix Concatenate3/2
  Matrix Concatenate2/1 -> Matrix Concatenate3/3
  Matrix Concatenate3/1 -> Out1/1
  cos(alpha)/1 -> Matrix Concatenate/1, Matrix Concatenate2/3
  Constant1/1 -> Matrix Concatenate/2, Matrix Concatenate1/1, Matrix Concatenate1/3, Matrix Concatenate2/2
  Constant/1 -> Matrix Concatenate1/2
  In1/1 -> cos(alpha)/1, sin(alpha)/1
  Gain/1 -> Matrix Concatenate/3
  sin(alpha)/1 -> Gain/1, Gain1/1
  Gain1/1 -> Matrix Concatenate2/1

== system fixed_wing_sim/A/C + Low Level Control /UAV Internal Closed Loops/UAV model/Aerodynamics Equations/F_WIND --> F_ABC/R_(alpha) ==
  note: cos  0  sin
      | 0    1    0
      | -sin   0  cos
  note: R_(-alpha) -->
  In1 : Inport
  Constant : Constant
  Constant1 : Constant  Value=0
  Gain : Gain  Gain=-1
  Gain1 : Gain
  Matrix Concatenate : Concatenate  NumInputs=3  Mode=Multidimensional array
  Matrix Concatenate1 : Concatenate  NumInputs=3  Mode=Multidimensional array
  Matrix Concatenate2 : Concatenate  NumInputs=3  Mode=Multidimensional array
  Matrix Concatenate3 : Concatenate  NumInputs=3  Mode=Multidimensional array  ConcatenateDimension=2
  cos(alpha) : Trigonometry  Operator=cos
  sin(alpha) : Trigonometry
  Out1 : Outport
  wires:
  Matrix Concatenate/1 -> Matrix Concatenate3/1
  Matrix Concatenate1/1 -> Matrix Concatenate3/2
  Matrix Concatenate2/1 -> Matrix Concatenate3/3
  Matrix Concatenate3/1 -> Out1/1
  cos(alpha)/1 -> Matrix Concatenate/1, Matrix Concatenate2/3
  Constant1/1 -> Matrix Concatenate/2, Matrix Concatenate1/1, Matrix Concatenate1/3, Matrix Concatenate2/2
  Constant/1 -> Matrix Concatenate1/2
  In1/1 -> cos(alpha)/1, sin(alpha)/1
  Gain/1 -> Matrix Concatenate/3
  sin(alpha)/1 -> Gain/1, Gain1/1
  Gain1/1 -> Matrix Concatenate2/1

== system fixed_wing_sim/A/C + Low Level Control /UAV Internal Closed Loops/UAV model/Aerodynamics Equations/F_WIND --> F_ABC/R_beta ==
  note: cos  sin   0
      | -sin  cos  0
      | 0       0     1
  note: R_(beta) -->
  In1 : Inport
  Constant : Constant
  Constant1 : Constant  Value=0
  Gain : Gain  Gain=-1
  Matrix Concatenate : Concatenate  NumInputs=3  Mode=Multidimensional array
  Matrix Concatenate1 : Concatenate  NumInputs=3  Mode=Multidimensional array
  Matrix Concatenate2 : Concatenate  NumInputs=3  Mode=Multidimensional array
  Matrix Concatenate3 : Concatenate  NumInputs=3  Mode=Multidimensional array  ConcatenateDimension=2
  cos(beta) : Trigonometry  Operator=cos
  sin(beta) : Trigonometry
  Out1 : Outport
  wires:
  Matrix Concatenate/1 -> Matrix Concatenate3/1
  Matrix Concatenate1/1 -> Matrix Concatenate3/2
  Matrix Concatenate2/1 -> Matrix Concatenate3/3
  Matrix Concatenate3/1 -> Out1/1
  cos(beta)/1 -> Matrix Concatenate/1, Matrix Concatenate1/2
  Gain/1 -> Matrix Concatenate/2
  sin(beta)/1 -> Gain/1, Matrix Concatenate1/1
  Constant1/1 -> Matrix Concatenate/3, Matrix Concatenate1/3, Matrix Concatenate2/1, Matrix Concatenate2/2
  Constant/1 -> Matrix Concatenate2/3
  In1/1 -> cos(beta)/1, sin(beta)/1

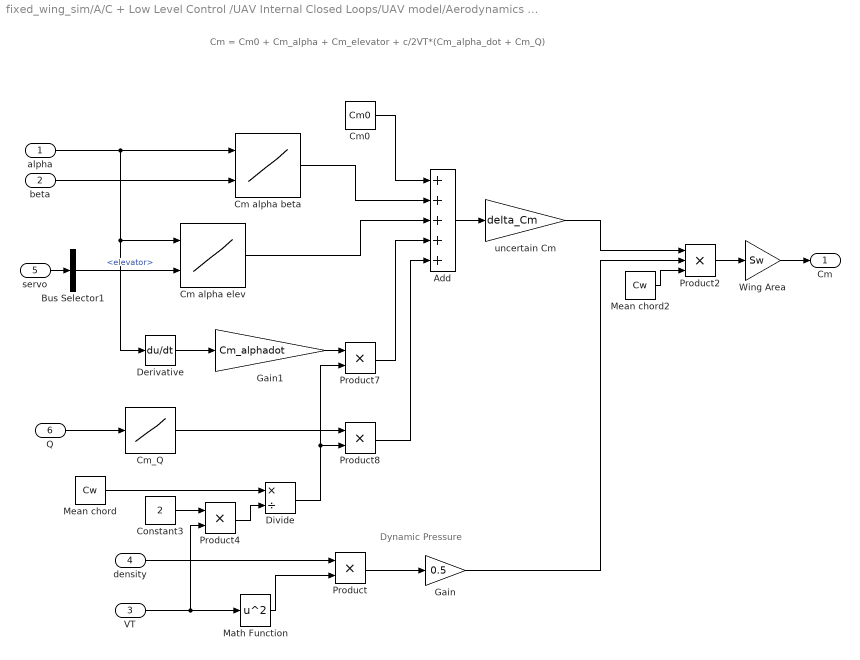
== system fixed_wing_sim/A/C + Low Level Control /UAV Internal Closed Loops/UAV model/Aerodynamics Equations/M_Aero_WIND/Pitching Moment ==
  note: Cm = Cm0 + Cm_alpha + Cm_elevator + c/2VT*(Cm_alpha_dot + Cm_Q)
  note: Dynamic Pressure
  alpha : Inport
  beta : Inport  Port=2
  VT : Inport  Port=3
  density : Inport  Port=4
  servo : Inport  Port=5
  Q : Inport  Port=6
  Add : Sum  Inputs=+++++
  Bus Selector1 : BusSelector  OutputSignals=elevator
  Cm alpha beta : Lookup_n-D  BreakpointsForDimension1=AlphaBnd  BreakpointsForDimension2=BetaBnd  Table=Cm_alpha_beta  RndMeth=Simplest  InputSameDT=on
  Cm alpha elev : Lookup_n-D  BreakpointsForDimension1=AlphaBnd  BreakpointsForDimension2=ElevBnd  Table=Cm_elev  RndMeth=Simplest  InputSameDT=on
  Cm0 : Constant  Value=Cm0
  Cm_Q : Lookup_n-D  NumberOfTableDimensions=1  BreakpointsForDimension1=QBnd  Table=Cm_Q  RndMeth=Simplest  InputSameDT=on
  Constant3 : Constant  Value=2
  Derivative : Derivative
  Divide : Product  Inputs=*/
  Gain : Gain  Gain=0.5
  Gain1 : Gain  Gain=Cm_alphadot
  Math Function : Math  Operator=square  SaturateOnIntegerOverflow=on
  Mean chord : Constant  Value=Cw
  Mean chord2 : Constant  Value=Cw
  Product{,4,7..8} (4 alike) : Product  RndMeth=Zero
  Product2 : Product  Inputs=3  RndMeth=Zero
  Wing Area : Gain  Gain=Sw
  uncertain Cm : Gain  Gain=delta_Cm
  Cm : Outport
  wires:
  VT/1 -> Math Function/1, Product4/2
  Wing Area/1 -> Cm/1
  Product/1 -> Gain/1
  Product2/1 -> Wing Area/1
  density/1 -> Product/1
  Math Function/1 -> Product/2
  Product4/1 -> Divide/2
  Mean chord/1 -> Divide/1
  Constant3/1 -> Product4/1
  Divide/1 -> Product7/2, Product8/2
  Gain/1 -> Product2/2
  Add/1 -> uncertain Cm/1
  Product7/1 -> Add/4
  Product8/1 -> Add/5
  servo/1 -> Bus Selector1/1
  Cm0/1 -> Add/1
  Gain1/1 -> Product7/1
  Derivative/1 -> Gain1/1
  Q/1 -> Cm_Q/1
  Cm_Q/1 -> Product8/1
  Mean chord2/1 -> Product2/3
  uncertain Cm/1 -> Product2/1
  Cm alpha beta/1 -> Add/2
  alpha/1 -> Cm alpha beta/1, Cm alpha elev/1, Derivative/1
  beta/1 -> Cm alpha beta/2
  Cm alpha elev/1 -> Add/3
  Bus Selector1/1 -> Cm alpha elev/2  "<elevator>"

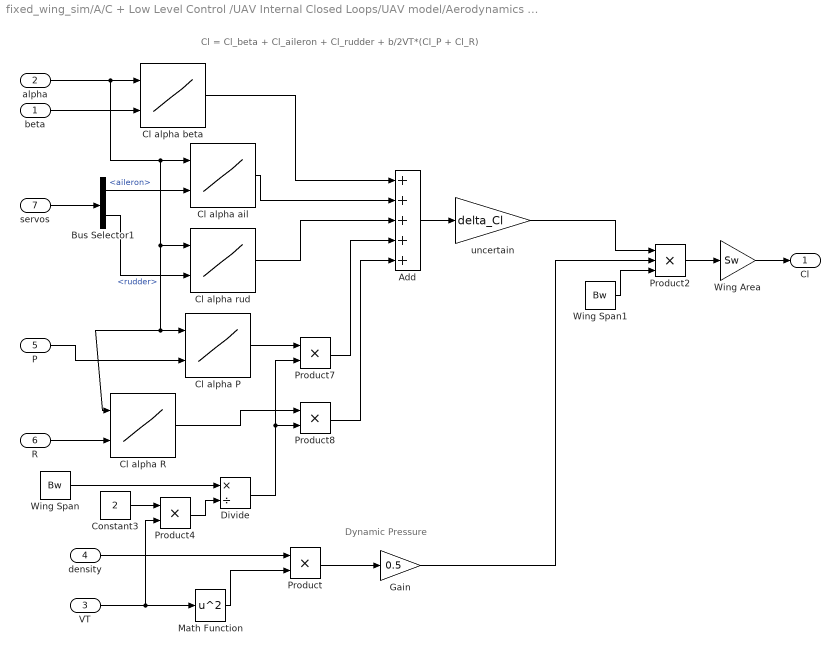
== system fixed_wing_sim/A/C + Low Level Control /UAV Internal Closed Loops/UAV model/Aerodynamics Equations/M_Aero_WIND/Rolling Moment ==
  note: Cl = Cl_beta + Cl_aileron + Cl_rudder + b/2VT*(Cl_P + Cl_R)
  note: Dynamic Pressure
  beta : Inport
  alpha : Inport  Port=2
  VT : Inport  Port=3
  density : Inport  Port=4
  P : Inport  Port=5
  R : Inport  Port=6
  servos : Inport  Port=7
  Add : Sum  Inputs=+++++
  Bus Selector1 : BusSelector  OutputSignals=aileron,rudder
  Cl alpha P : Lookup_n-D  BreakpointsForDimension1=AlphaBnd  BreakpointsForDimension2=PBnd  Table=Cl_P  RndMeth=Simplest  InputSameDT=on
  Cl alpha R : Lookup_n-D  BreakpointsForDimension1=AlphaBnd  BreakpointsForDimension2=RBnd  Table=Cl_R  RndMeth=Simplest  InputSameDT=on
  Cl alpha ail : Lookup_n-D  BreakpointsForDimension1=AlphaBnd  BreakpointsForDimension2=AilBnd  Table=Cl_ail  RndMeth=Simplest  InputSameDT=on
  Cl alpha beta : Lookup_n-D  BreakpointsForDimension1=AlphaBnd  BreakpointsForDimension2=BetaBnd  Table=Cl_alpha_beta  RndMeth=Simplest  InputSameDT=on
  Cl alpha rud : Lookup_n-D  BreakpointsForDimension1=AlphaBnd  BreakpointsForDimension2=RudBnd  Table=Cl_rud  RndMeth=Simplest  InputSameDT=on
  Constant3 : Constant  Value=2
  Divide : Product  Inputs=*/
  Gain : Gain  Gain=0.5
  Math Function : Math  Operator=square  SaturateOnIntegerOverflow=on
  Product{,4,7..8} (4 alike) : Product  RndMeth=Zero
  Product2 : Product  Inputs=3  RndMeth=Zero
  Wing Area : Gain  Gain=Sw
  Wing Span : Constant  Value=Bw
  Wing Span1 : Constant  Value=Bw
  uncertain : Gain  Gain=delta_Cl
  Cl : Outport
  wires:
  VT/1 -> Math Function/1, Product4/2
  Wing Area/1 -> Cl/1
  Product/1 -> Gain/1
  Add/1 -> uncertain/1
  Product2/1 -> Wing Area/1
  density/1 -> Product/1
  Math Function/1 -> Product/2
  Product4/1 -> Divide/2
  Wing Span/1 -> Divide/1
  Constant3/1 -> Product4/1
  Divide/1 -> Product8/2, Product7/2
  Product7/1 -> Add/4
  Product8/1 -> Add/5
  Gain/1 -> Product2/2
  Cl alpha ail/1 -> Add/2
  servos/1 -> Bus Selector1/1
  Bus Selector1/1 -> Cl alpha ail/2  "<aileron>"
  P/1 -> Cl alpha P/2
  R/1 -> Cl alpha R/2
  Wing Span1/1 -> Product2/3
  uncertain/1 -> Product2/1
  alpha/1 -> Cl alpha beta/1, Cl alpha ail/1, Cl alpha P/1, Cl alpha R/1, Cl alpha rud/1
  beta/1 -> Cl alpha beta/2
  Cl alpha beta/1 -> Add/1
  Cl alpha P/1 -> Product7/1
  Cl alpha R/1 -> Product8/1
  Bus Selector1/2 -> Cl alpha rud/2  "<rudder>"
  Cl alpha rud/1 -> Add/3

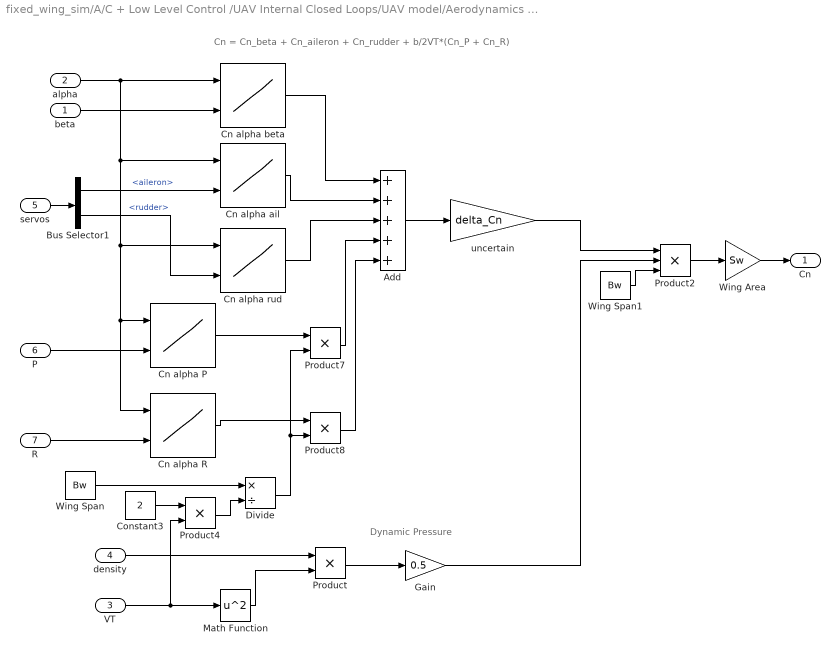
== system fixed_wing_sim/A/C + Low Level Control /UAV Internal Closed Loops/UAV model/Aerodynamics Equations/M_Aero_WIND/Yawing Moment ==
  note: Cn = Cn_beta + Cn_aileron + Cn_rudder + b/2VT*(Cn_P + Cn_R)
  note: Dynamic Pressure
  beta : Inport
  alpha : Inport  Port=2
  VT : Inport  Port=3
  density : Inport  Port=4
  servos : Inport  Port=5
  P : Inport  Port=6
  R : Inport  Port=7
  Add : Sum  Inputs=+++++
  Bus Selector1 : BusSelector  OutputSignals=aileron,rudder
  Cn alpha P : Lookup_n-D  BreakpointsForDimension1=AlphaBnd  BreakpointsForDimension2=PBnd  Table=Cn_P  RndMeth=Simplest  InputSameDT=on
  Cn alpha R : Lookup_n-D  BreakpointsForDimension1=AlphaBnd  BreakpointsForDimension2=RBnd  Table=Cn_R  RndMeth=Simplest  InputSameDT=on
  Cn alpha ail : Lookup_n-D  BreakpointsForDimension1=AlphaBnd  BreakpointsForDimension2=AilBnd  Table=Cn_ail  RndMeth=Simplest  InputSameDT=on
  Cn alpha beta : Lookup_n-D  BreakpointsForDimension1=AlphaBnd  BreakpointsForDimension2=BetaBnd  Table=Cn_alpha_beta  RndMeth=Simplest  InputSameDT=on
  Cn alpha rud : Lookup_n-D  BreakpointsForDimension1=AlphaBnd  BreakpointsForDimension2=RudBnd  Table=Cn_rud  RndMeth=Simplest  InputSameDT=on
  Constant3 : Constant  Value=2
  Divide : Product  Inputs=*/
  Gain : Gain  Gain=0.5
  Math Function : Math  Operator=square  SaturateOnIntegerOverflow=on
  Product{,4,7..8} (4 alike) : Product  RndMeth=Zero
  Product2 : Product  Inputs=3  RndMeth=Zero
  Wing Area : Gain  Gain=Sw
  Wing Span : Constant  Value=Bw
  Wing Span1 : Constant  Value=Bw
  uncertain : Gain  Gain=delta_Cn
  Cn : Outport
  wires:
  VT/1 -> Math Function/1, Product4/2
  Wing Area/1 -> Cn/1
  Product/1 -> Gain/1
  Add/1 -> uncertain/1
  Product2/1 -> Wing Area/1
  density/1 -> Product/1
  Math Function/1 -> Product/2
  Product4/1 -> Divide/2
  Wing Span/1 -> Divide/1
  Constant3/1 -> Product4/1
  Divide/1 -> Product8/2, Product7/2
  Product7/1 -> Add/4
  Product8/1 -> Add/5
  Gain/1 -> Product2/2
  servos/1 -> Bus Selector1/1
  Bus Selector1/1 -> Cn alpha ail/2  "<aileron>"
  Cn alpha ail/1 -> Add/2
  P/1 -> Cn alpha P/2
  R/1 -> Cn alpha R/2
  Wing Span1/1 -> Product2/3
  uncertain/1 -> Product2/1
  Cn alpha beta/1 -> Add/1
  alpha/1 -> Cn alpha beta/1, Cn alpha ail/1, Cn alpha P/1, Cn alpha R/1, Cn alpha rud/1
  beta/1 -> Cn alpha beta/2
  Cn alpha P/1 -> Product7/1
  Cn alpha R/1 -> Product8/1
  Cn alpha rud/1 -> Add/3
  Bus Selector1/2 -> Cn alpha rud/2  "<rudder>"

== system fixed_wing_sim/A/C + Low Level Control /UAV Internal Closed Loops/UAV model/Body-Axes 6DOF Equations/Force Equations/NED --> ABC ==
  note: ABC = R_phi * R_theta * R_psi * NED
  attitude : Inport
  NED : Inport  Port=2
  Bus Selector : BusSelector  OutputSignals=phi,theta,psi
  Product : Product  Multiplication=Matrix(*)  RndMeth=Zero
  Product1 : Product  Multiplication=Matrix(*)  RndMeth=Zero
  Product2 : Product  Multiplication=Matrix(*)  RndMeth=Zero
  "R_phi " : Subsystem
  R_psi : Subsystem
  R_theta : Subsystem
  ABC : Outport
  wires:
  attitude/1 -> Bus Selector/1
  R_theta/1(Out1) -> Product/2
  Product/1 -> Product1/1
  Bus Selector/1 -> "R_phi "/1(In1)  "<phi>"
  "R_phi "/1(Out1) -> Product/1
  R_psi/1(Out1) -> Product1/2
  Product1/1 -> Product2/1
  NED/1 -> Product2/2
  Product2/1 -> ABC/1
  Bus Selector/2 -> R_theta/1(In1)  "<theta>"
  Bus Selector/3 -> R_psi/1(In1)  "<psi>"

== system fixed_wing_sim/A/C + Low Level Control /UAV Internal Closed Loops/UAV model/Body-Axes 6DOF Equations/Force Equations/Vector Product ==
  V1 : Inport
  V2 : Inport  Port=2
  Mux : Mux  Inputs=2
  Mux1 : Mux  Inputs=3
  i : Fcn  Expr=u(2)*u(6) - u(3)*u(5)
  j : Fcn  Expr=u(3)*u(4) - u(1)*u(6)
  k : Fcn  Expr=u(1)*u(5) - u(2)*u(4)
  V1 x V2 : Outport
  wires:
  V1/1 -> Mux/1
  V2/1 -> Mux/2
  Mux/1 -> i/1, j/1, k/1
  i/1 -> Mux1/1
  j/1 -> Mux1/2
  k/1 -> Mux1/3
  Mux1/1 -> V1 x V2/1

== system fixed_wing_sim/A/C + Low Level Control /UAV Internal Closed Loops/UAV model/Body-Axes 6DOF Equations/Moment Equations/Inertia ==
  Constant : Constant  Value=Jx
  Constant1 : Constant  Value=Jy
  Constant2 : Constant  Value=Jz
  Constant3 : Constant  Value=-Jxz
  Constant4 : Constant  Value=0
  Matrix Concatenation10 : Concatenate  NumInputs=3  Mode=Multidimensional array
  Matrix Concatenation11 : Concatenate  NumInputs=3  Mode=Multidimensional array  ConcatenateDimension=2
  Matrix Concatenation8 : Concatenate  NumInputs=3  Mode=Multidimensional array
  Matrix Concatenation9 : Concatenate  NumInputs=3  Mode=Multidimensional array
  J_b : Outport
  wires:
  Matrix Concatenation8/1 -> Matrix Concatenation11/1
  Matrix Concatenation9/1 -> Matrix Concatenation11/2
  Matrix Concatenation10/1 -> Matrix Concatenation11/3
  Matrix Concatenation11/1 -> J_b/1
  Constant/1 -> Matrix Concatenation8/1
  Constant4/1 -> Matrix Concatenation8/2, Matrix Concatenation9/1, Matrix Concatenation9/3, Matrix Concatenation10/2
  Constant3/1 -> Matrix Concatenation8/3, Matrix Concatenation10/1
  Constant1/1 -> Matrix Concatenation9/2
  Constant2/1 -> Matrix Concatenation10/3
